simulink model "PLANTA_CONTROL_OBS"  (R2024b)
settings: Solver=FixedStepAuto  StartTime=0.0  StopTime=inf  FixedStep=0.001  MaxStep=0.0005  RelTol=1e-4
InitFcn:
  | load('ml_breakpoints.mat')
  | load('l_breakpoints.mat')
  | load('at_breakpoints.mat')
  | load('Kp_table.mat')
  | load('Kd_table.mat')
undefined symbols (not defined in the file): A_hm, A_tm, at_breakpoints, at_max, b_ha, B_hm, b_ta, B_tm, bcx, bcy, bhd, bhEb, bhm, bt, btd, btm, btw, bwu, C_hm, C_tm, D_hm, D_tm, DiscIntNeverNeededParam, dl_h_ini, dx_l_ini, dx_t_ini, dx_td_ini, dxt_max, dy_l_ini, F01_a_t_max, F01_Ts1, F02_a_h_max, F02_Ts1, F03_a_h_max, F03_a_t_max, F03_dxt_max, F03_Ts1, Fhw_min, g, Hc, ih, it, Jhd_hEb, Jhm_hb, Jtd, Jtm_tb, K_hsa, K_hsia, K_tsa, K_tsia, Kcy, Kd_table, Ke_tita, Ke_w, kp_pos, Kp_table, kp_w, Ktw, kwu, l_breakpoints ... (+26)
libraries: simulink x7, spsEdgeDetectorLib x5, simulink_extras x2, dspsigops x2, vrlib x1, dspstat3 x1
(part 3 of 4)

== system PLANTA_CONTROL_OBS/Masa contenedor ==
  Fwh : Inport
  TLK : Inport  Port=2
  Edge Detector : spsEdgeDetectorLib/Edge Detector  model=Falling  ic=0  Ts=-1
      settings: LibrarySourceBlock=sps_lib/Control/Edge Detector
  Edge Detector1 : spsEdgeDetectorLib/Edge Detector  model=Rising  ic=0  Ts=-1
      settings: LibrarySourceBlock=sps_lib/Control/Edge Detector
  Gain8 : Gain  Gain=2/g
  Product : Product
  S-R Flip-Flop : simulink_extras/Flip Flops/S-R Flip-Flop  initial_condition=0
  Unit Delay : UnitDelay  SampleTime=-1  HasFrameUpgradeWarning=on
  Mc_X : Outport
  wires:
  TLK/1 -> Unit Delay/1
  Edge Detector/1 -> S-R Flip-Flop/2
  Edge Detector1/1 -> S-R Flip-Flop/1
  S-R Flip-Flop/1 -> Product/2
  Product/1 -> Mc_X/1
  Unit Delay/1 -> Edge Detector1/1, Edge Detector/1
  Fwh/1 -> Gain8/1  "m estimada"
  Gain8/1 -> Product/1  "m estimada"

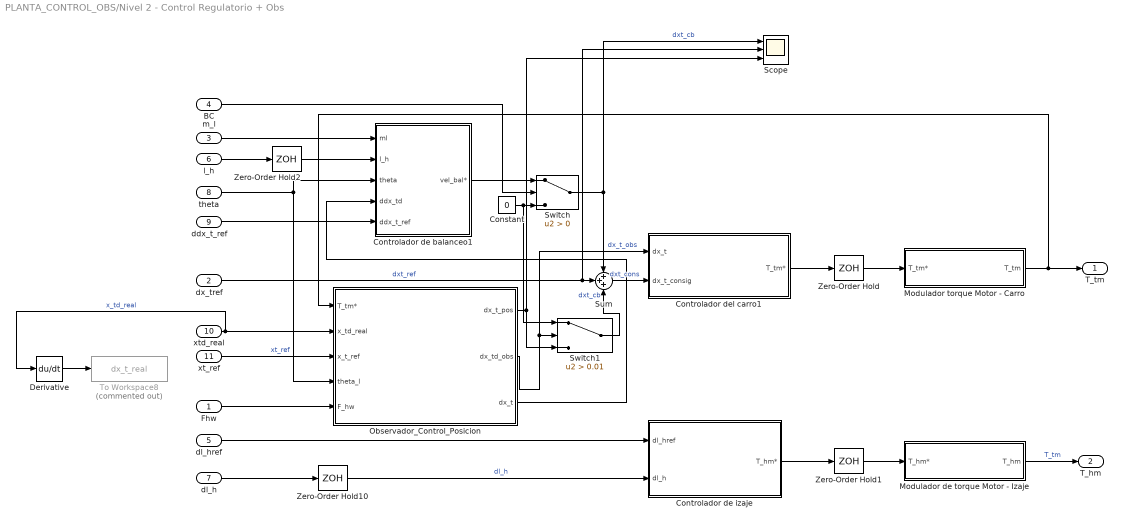
== system PLANTA_CONTROL_OBS/Nivel 2 - Control Regulatorio + Obs ==
  Fhw : Inport
  dx_tref : Inport  Port=2
  m_l : Inport  Port=3
  BC : Inport  Port=4
  dl_href : Inport  Port=5
  l_h : Inport  Port=6
  dl_h : Inport  Port=7
  theta : Inport  Port=8
  ddx_t_ref : Inport  Port=9
  xtd_real : Inport  Port=10
  xt_ref : Inport  Port=11
  Constant : Constant  Value=0
  Controlador de balanceo1 : Subsystem
  Controlador de izaje : Subsystem
  Controlador del carro1 : Subsystem
  Derivative : Derivative
  Modulador de torque Motor - Izaje : Subsystem
  Modulador torque Motor - Carro : Subsystem
  Observador_Control_Posicion : Subsystem
  Scope : Scope  NumInputPorts=3
  Sum : Sum  Inputs=+++
  Switch : Switch  Criteria=u2 > Threshold  SaturateOnIntegerOverflow=off  InputSameDT=off
  Switch1 : Switch  Criteria=u2 > Threshold  Threshold=0.01  SaturateOnIntegerOverflow=off  InputSameDT=off
  To Workspace8 : ToWorkspace  Commented=on  VariableName=dx_t_real  SaveFormat=Timeseries  SampleTime=-1
      settings: Save2DSignal=2-D array (concatenate along first dimension)
  Zero-Order Hold{,1..2,10} (4 alike) : ZeroOrderHold  SampleTime=T_s2
  T_tm : Outport
  T_hm : Outport  Port=2
  wires:
  Zero-Order Hold1/1 -> Modulador de torque Motor - Izaje/1(T_hm*)
  dl_h/1 -> Zero-Order Hold10/1
  Controlador de izaje/1(T_hm*) -> Zero-Order Hold1/1
  Modulador de torque Motor - Izaje/1(T_hm) -> T_hm/1  "T_tm"
  Zero-Order Hold/1 -> Modulador torque Motor - Carro/1(T_tm*)
  Modulador torque Motor - Carro/1(T_tm) -> Observador_Control_Posicion/1(T_tm*), T_tm/1
  l_h/1 -> Zero-Order Hold2/1
  Constant/1 -> Switch1/1, Switch/3
  m_l/1 -> Controlador de balanceo1/1(ml)
  BC/1 -> Switch/2
  Controlador del carro1/1(T_tm*) -> Zero-Order Hold/1
  Controlador de balanceo1/1(vel_bal*) -> Switch/1
  theta/1 -> Controlador de balanceo1/3(theta), Observador_Control_Posicion/4(theta_l)
  dx_tref/1 -> Scope/2, Sum/2  "dxt_ref"
  Sum/1 -> Controlador del carro1/2(dx_t_consig)  "dxt_cons"
  Switch/1 -> Scope/1, Sum/1  "dxt_cb"
  ddx_t_ref/1 -> Controlador de balanceo1/5(ddx_t_ref)
  Observador_Control_Posicion/1(dx_t_pos) -> Switch1/3, Scope/3
  xtd_real/1 -> Derivative/1, Observador_Control_Posicion/2(x_td_real)  "x_td_real"
  xt_ref/1 -> Observador_Control_Posicion/3(x_t_ref)  "xt_ref"
  Fhw/1 -> Observador_Control_Posicion/5(F_hw)
  Observador_Control_Posicion/2(dx_td_obs) -> Switch1/2, Controlador del carro1/1(dx_t)  "dx_t_obs"
  Zero-Order Hold10/1 -> Controlador de izaje/2(dl_h)  "dl_h"
  dl_href/1 -> Controlador de izaje/1(dl_href)
  Zero-Order Hold2/1 -> Controlador de balanceo1/2(l_h)
  Switch1/1 -> Sum/3  "dxt_cb"
  Derivative/1 -> To Workspace8/1
  Observador_Control_Posicion/3(dx_t) -> Controlador de balanceo1/4(ddx_td)

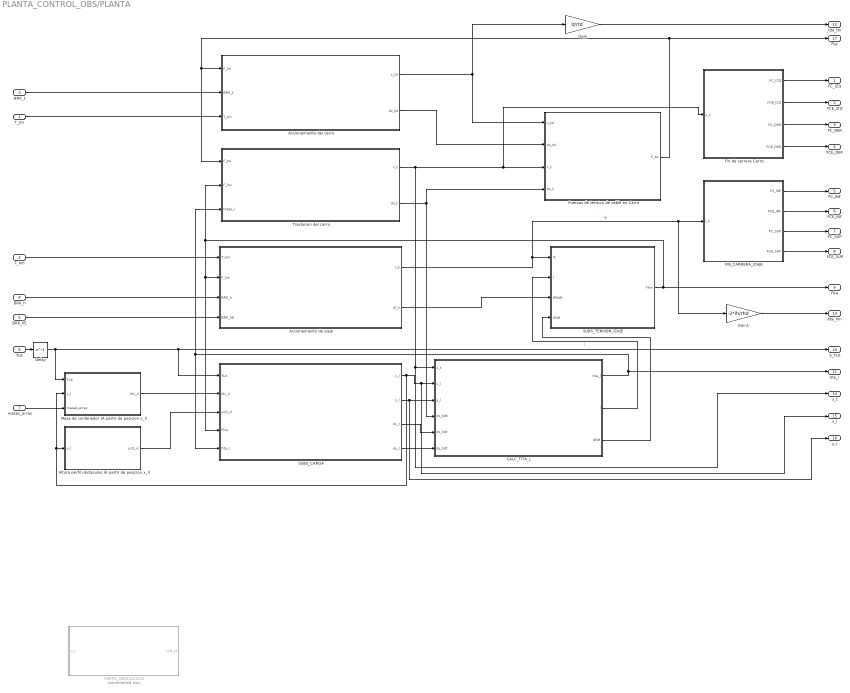
== system PLANTA_CONTROL_OBS/PLANTA ==
  T_tm : Inport
  T_hm : Inport  Port=2
  BRK_t : Inport  Port=3
  BRK_h : Inport  Port=4
  BRK_hE : Inport  Port=5
  TLK : Inport  Port=6
  masas_array : Inport  Port=7
  Accionamiento de Izaje : Subsystem
  Accionamiento del carro : Subsystem
  Altura perfil obstaculos (A partir de posicion x_l) : Subsystem
  CALC_TITA_L : Subsystem
  Delay : Delay  DelayLength=1  InputProcessing=Columns as channels (frame based)  SampleTime=T_s1
  FIN_CARRERA_IZAJE : Subsystem
  Fin de carrera Carro : Subsystem
  Fuerzas de tension de cable en Carro : Subsystem
  Gain : Gain  Gain=it/rtd
  Gain1 : Gain  Gain=-2*ih/rhd
  Masa de contenedor (A partir de posicion x_l) : Subsystem
  PERFIL_OBSTACULOS : Subsystem  Commented=on
  SUBS_CARGA : Subsystem
  SUBS_TENSION_IZAJE : Subsystem
  Traslacion del carro : Subsystem
  FC_IZQ : Outport
  FCE_IZQ : Outport  Port=2
  FC_DER : Outport  Port=3
  FCE_DER : Outport  Port=4
  FC_INF : Outport  Port=5
  FCE_INF : Outport  Port=6
  FC_SUP : Outport  Port=7
  FCE_SUP : Outport  Port=8
  Fhw : Outport  Port=9
  S_TLK : Outport  Port=10
  tita_l : Outport  Port=11
  tita_tm : Outport  Port=12
  tita_hm : Outport  Port=13
  x_t : Outport  Port=14
  x_l : Outport  Port=15
  y_l : Outport  Port=16
  Ftw : Outport  Port=17
  wires:
  Gain/1 -> tita_tm/1
  Traslacion del carro/2(dx_t) -> CALC_TITA_L/4(dx_t/dt), Fuerzas de tension de cable en Carro/4(dx_t)
  SUBS_TENSION_IZAJE/1(Fhw) -> Fhw/1, Traslacion del carro/2(F_hw), Accionamiento de Izaje/2(F_hw), SUBS_CARGA/4(Fhw)
  CALC_TITA_L/3(dl/dt) -> SUBS_TENSION_IZAJE/4(dl/dt)
  BRK_h/1 -> Accionamiento de Izaje/3(BRK_h)
  TLK/1 -> Delay/1
  BRK_t/1 -> Accionamiento del carro/2(BRK_t)
  Accionamiento del carro/1(x_td) -> Gain/1, Fuerzas de tension de cable en Carro/1(x_td)
  BRK_hE/1 -> Accionamiento de Izaje/4(BRK_hE)
  Accionamiento del carro/2(dx_td) -> Fuerzas de tension de cable en Carro/2(dx_td)
  FIN_CARRERA_IZAJE/3(FC_SUP) -> FC_SUP/1
  Fin de carrera Carro/4(FCE_DER) -> FCE_DER/1
  SUBS_CARGA/4(dy_l) -> CALC_TITA_L/6(dy_l/dt)
  CALC_TITA_L/2(l) -> SUBS_TENSION_IZAJE/2(l)  "l"
  Fuerzas de tension de cable en Carro/1(F_tw) -> Ftw/1, Accionamiento del carro/1(F_tw), Traslacion del carro/1(F_tw)
  SUBS_CARGA/3(dx_l) -> CALC_TITA_L/5(dx_l/dt)
  Altura perfil obstaculos (A partir de posicion x_l)/1(yc0_xl) -> SUBS_CARGA/3(yc0_xl)
  Accionamiento de Izaje/1(l_h) -> SUBS_TENSION_IZAJE/1(Ih), FIN_CARRERA_IZAJE/1(l_h), Gain1/1  "lh"
  Accionamiento de Izaje/2(dl_h) -> SUBS_TENSION_IZAJE/3(dlh/dt)
  T_tm/1 -> Accionamiento del carro/3(T_tm)
  Fin de carrera Carro/2(FCE_IZQ) -> FCE_IZQ/1
  T_hm/1 -> Accionamiento de Izaje/1(T_hm)
  FIN_CARRERA_IZAJE/1(FC_INF) -> FC_INF/1
  Gain1/1 -> tita_hm/1
  FIN_CARRERA_IZAJE/2(FCE_INF) -> FCE_INF/1
  Fin de carrera Carro/1(FC_IZQ) -> FC_IZQ/1
  FIN_CARRERA_IZAJE/4(FCE_SUP) -> FCE_SUP/1
  Fin de carrera Carro/3(FC_DER) -> FC_DER/1
  SUBS_CARGA/1(x_l) -> Masa de contenedor (A partir de posicion x_l)/2(x_l), Altura perfil obstaculos (A partir de posicion x_l)/1(x_l), x_l/1, CALC_TITA_L/2(x_l)
  CALC_TITA_L/1(tita_l) -> tita_l/1, Traslacion del carro/3(theta_l), SUBS_CARGA/5(tita_l)
  Traslacion del carro/1(x_t) -> CALC_TITA_L/1(x_t), x_t/1, Fin de carrera Carro/1(x_t), Fuerzas de tension de cable en Carro/3(x_t)
  SUBS_CARGA/2(y_l) -> y_l/1, CALC_TITA_L/3(y_l)
  Masa de contenedor (A partir de posicion x_l)/1(Mc_X) -> SUBS_CARGA/2(Mc_X)
  Delay/1 -> Masa de contenedor (A partir de posicion x_l)/1(TLK), S_TLK/1, SUBS_CARGA/1(TLK)
  masas_array/1 -> Masa de contenedor (A partir de posicion x_l)/3(masas_array)

== system PLANTA_CONTROL_OBS/Actualizar perfil/Enabled Subsystem ==
  index : Inport
  Enable : EnablePort
  Actualiza perfil : MATLAB Function  TreatAsAtomicUnit=on
  Constant16 : Constant  Value=Hc
  Data Store Read3 : DataStoreRead  DataStoreName=y0_global  IndexOptions=Index vector (dialog)  Indices=1  OutputSizes=1
  y0_actualizado : Outport
  wires:
  Data Store Read3/1 -> Actualiza perfil/2(y0)
  Constant16/1 -> Actualiza perfil/3(Hc)
  index/1 -> Actualiza perfil/1(index)
  Actualiza perfil/1(y0_actualizado) -> y0_actualizado/1

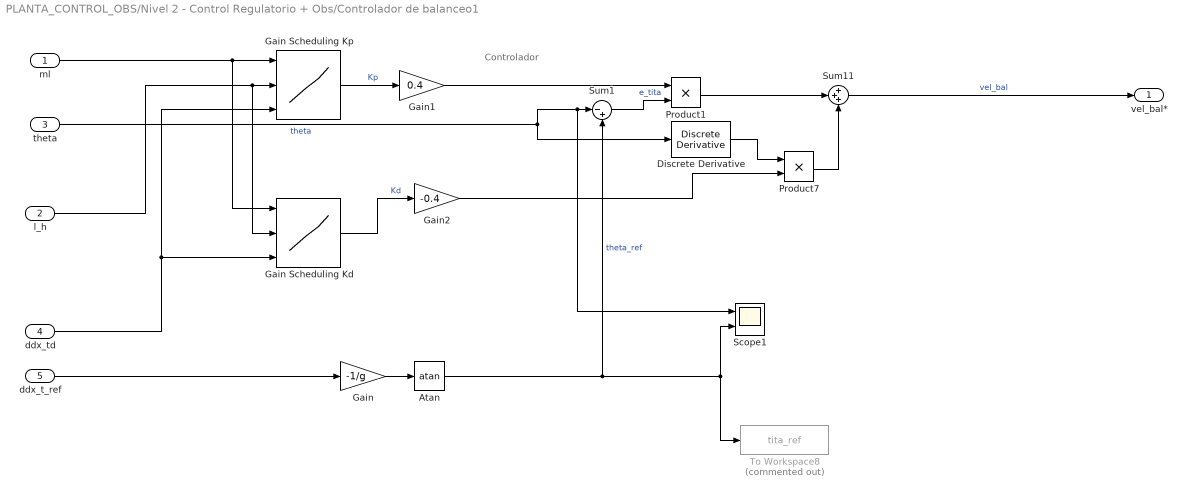
== system PLANTA_CONTROL_OBS/Nivel 2 - Control Regulatorio + Obs/Controlador de balanceo1 ==
  note: Controlador
  ml : Inport
  l_h : Inport  Port=2
  theta : Inport  Port=3
  ddx_td : Inport  Port=4
  ddx_t_ref : Inport  Port=5
  Atan : Trigonometry  Operator=atan
  Discrete Derivative : simulink/Discrete/Discrete Derivative  gainval=1.0  ICPrevScaledInput=0.0  OutMin=[]  OutMax=[]  OutDataType=fixdt(1, 16)  OutScaling=2^-10  DoSatur=off
  Gain : Gain  Gain=-1/g
  Gain Scheduling Kd : Lookup_n-D  NumberOfTableDimensions=3  BreakpointsForDimension1=ml_breakpoints  BreakpointsForDimension2=l_breakpoints  BreakpointsForDimension3=at_breakpoints  BreakpointsForDimension4=at_breakpoints  Table=Kd_table  InterpMethod=Flat  ExtrapMethod=Clip  InternalRulePriority=Speed  RndMeth=Simplest
      settings: InputPortMap=u0,u1,u2
  Gain Scheduling Kp : Lookup_n-D  NumberOfTableDimensions=3  BreakpointsForDimension1=ml_breakpoints  BreakpointsForDimension2=l_breakpoints  BreakpointsForDimension3=at_breakpoints  BreakpointsForDimension4=at_breakpoints  Table=Kp_table  InterpMethod=Flat  ExtrapMethod=Clip  InternalRulePriority=Speed  RndMeth=Simplest
      settings: InputPortMap=u0,u1,u2
  Gain1 : Gain  Gain=0.4
  Gain2 : Gain  Gain=-0.4
  Product1 : Product
  Product7 : Product
  Scope1 : Scope  NumInputPorts=2
  Sum1 : Sum  Inputs=|-+
  Sum11 : Sum  Inputs=+++
  To Workspace8 : ToWorkspace  Commented=on  VariableName=tita_ref  SaveFormat=Timeseries  SampleTime=-1
      settings: Save2DSignal=2-D array (concatenate along first dimension)
  vel_bal* : Outport
  wires:
  Discrete Derivative/1 -> Product7/1
  Gain Scheduling Kd/1 -> Gain2/1  "Kd"
  Gain/1 -> Atan/1
  Gain Scheduling Kp/1 -> Gain1/1  "Kp"
  theta/1 -> Scope1/1, Sum1/1, Discrete Derivative/1  "theta"
  Product1/1 -> Sum11/2
  Atan/1 -> To Workspace8/1, Scope1/2, Sum1/2  "theta_ref"
  Product7/1 -> Sum11/3
  ddx_t_ref/1 -> Gain/1
  Sum1/1 -> Product1/2  "e_tita"
  Sum11/1 -> vel_bal*/1  "vel_bal"
  ml/1 -> Gain Scheduling Kd/1, Gain Scheduling Kp/1
  l_h/1 -> Gain Scheduling Kd/2, Gain Scheduling Kp/2
  Gain1/1 -> Product1/1
  Gain2/1 -> Product7/2
  ddx_td/1 -> Gain Scheduling Kd/3, Gain Scheduling Kp/3

== system PLANTA_CONTROL_OBS/Nivel 2 - Control Regulatorio + Obs/Controlador de izaje ==
  dl_href : Inport
  dl_h : Inport  Port=2
  Discrete-Time Integrator : DiscreteIntegrator  SampleTime=T_s2  ICPrevOutput=DiscIntNeverNeededParam  ICPrevScaledInput=DiscIntNeverNeededParam
  Discrete-Time Integrator1 : DiscreteIntegrator  SampleTime=T_s2  ICPrevOutput=DiscIntNeverNeededParam  ICPrevScaledInput=DiscIntNeverNeededParam
  Gain1 : Gain  Gain=K_hsia
  Gain2 : Gain  Gain=b_ha
  Gain8 : Gain  Gain=K_hsa
  Sum : Sum  Inputs=|+-
  Sum5 : Sum  Inputs=+|+|+
  T_hm* : Outport
  wires:
  Gain2/1 -> Sum5/3
  dl_h/1 -> Sum/2
  Sum5/1 -> T_hm*/1
  dl_href/1 -> Sum/1
  Gain1/1 -> Sum5/1
  Sum/1 -> Gain2/1, Discrete-Time Integrator/1  "d_ek"
  Gain8/1 -> Sum5/2
  Discrete-Time Integrator/1 -> Gain8/1, Discrete-Time Integrator1/1
  Discrete-Time Integrator1/1 -> Gain1/1

== system PLANTA_CONTROL_OBS/Nivel 2 - Control Regulatorio + Obs/Controlador del carro1 ==
  dx_t : Inport
  dx_t_consig : Inport  Port=2
  Discrete-Time Integrator : DiscreteIntegrator  SampleTime=T_s2  ICPrevOutput=DiscIntNeverNeededParam  ICPrevScaledInput=DiscIntNeverNeededParam
  Discrete-Time Integrator1 : DiscreteIntegrator  SampleTime=T_s2  ICPrevOutput=DiscIntNeverNeededParam  ICPrevScaledInput=DiscIntNeverNeededParam
  Gain1 : Gain  Gain=b_ta
  Gain2 : Gain  Gain=K_tsa
  Gain4 : Gain  Gain=K_tsia
  Sum : Sum  Inputs=|+-
  Sum5 : Sum  Inputs=+|+|+
  T_tm* : Outport
  wires:
  Sum/1 -> Discrete-Time Integrator/1, Gain1/1  "d_ek"
  dx_t_consig/1 -> Sum/1
  Sum5/1 -> T_tm*/1
  dx_t/1 -> Sum/2
  Gain2/1 -> Sum5/2
  Gain1/1 -> Sum5/3
  Gain4/1 -> Sum5/1
  Discrete-Time Integrator/1 -> Gain2/1, Discrete-Time Integrator1/1
  Discrete-Time Integrator1/1 -> Gain4/1

== system PLANTA_CONTROL_OBS/Nivel 2 - Control Regulatorio + Obs/Modulador de torque Motor - Izaje ==
  T_hm* : Inport
  State-Space : StateSpace  A=A_hm  B=B_hm  C=C_hm  D=D_hm  InitialCondition=0
  T_hm : Outport
  wires:
  T_hm*/1 -> State-Space/1
  State-Space/1 -> T_hm/1

== system PLANTA_CONTROL_OBS/Nivel 2 - Control Regulatorio + Obs/Modulador torque Motor - Carro ==
  T_tm* : Inport
  State-Space : StateSpace  A=A_tm  B=B_tm  C=C_tm  D=D_tm  InitialCondition=0
  T_tm : Outport
  wires:
  State-Space/1 -> T_tm/1
  T_tm*/1 -> State-Space/1

== system PLANTA_CONTROL_OBS/Nivel 2 - Control Regulatorio + Obs/Observador_Control_Posicion ==
  T_tm* : Inport
  x_td_real : Inport  Port=2
  x_t_ref : Inport  Port=3
  theta_l : Inport  Port=4
  F_hw : Inport  Port=5
  Discrete Derivative : simulink/Discrete/Discrete Derivative  gainval=1.0  ICPrevScaledInput=0.0  OutMin=[]  OutMax=[]  OutDataType=fixdt(1, 16)  OutScaling=2^-10  DoSatur=off
  Fuerzas de tension de cable en Carro : Subsystem
  Observador : Subsystem
  Subsystem : Subsystem
  Traslacion del carro : Subsystem
  dx_t_pos : Outport
  dx_td_obs : Outport  Port=2
  dx_t : Outport  Port=3
  wires:
  Observador/1(dx_td_obs) -> Fuerzas de tension de cable en Carro/2(dx_td), dx_td_obs/1  "dx_td_obs"
  x_td_real/1 -> Fuerzas de tension de cable en Carro/1(x_td), Observador/1(x_td)
  x_t_ref/1 -> Subsystem/2(xt_ref)
  Subsystem/1(dxt_pos) -> dx_t_pos/1
  Traslacion del carro/1(x_t) -> Fuerzas de tension de cable en Carro/3(x_t), Subsystem/1(xt_obs)  "x_t_obs"
  Traslacion del carro/2(dx_t) -> Fuerzas de tension de cable en Carro/4(dx_t), Discrete Derivative/1  "dx_t_obs"
  theta_l/1 -> Traslacion del carro/3(theta_l)
  F_hw/1 -> Traslacion del carro/2(F_hw)
  Fuerzas de tension de cable en Carro/1(F_tw) -> Traslacion del carro/1(F_tw)
  T_tm*/1 -> Observador/2(T_tm*)
  Discrete Derivative/1 -> dx_t/1

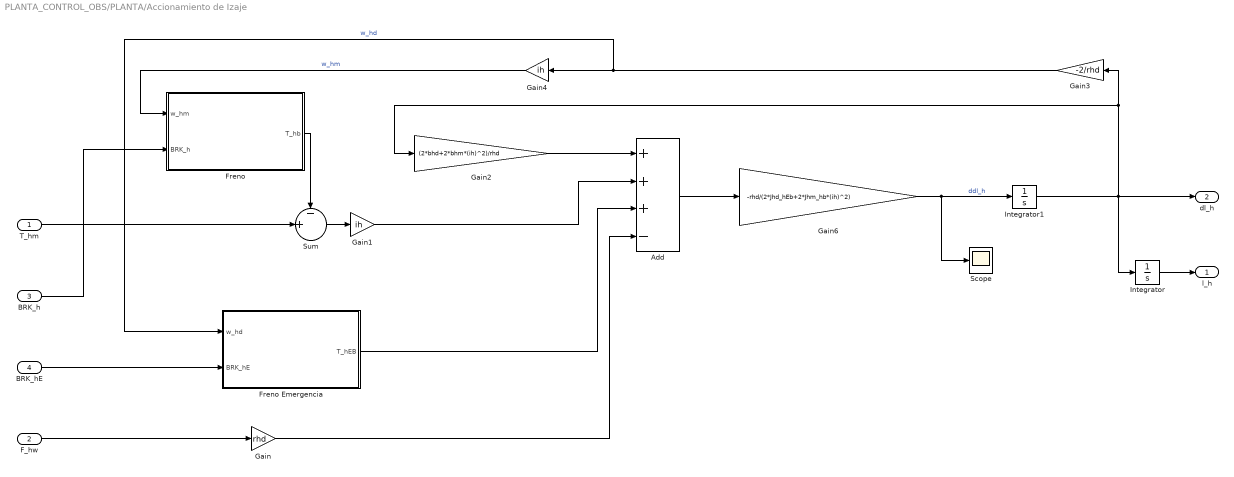
== system PLANTA_CONTROL_OBS/PLANTA/Accionamiento de Izaje ==
  T_hm : Inport
  F_hw : Inport  Port=2
  BRK_h : Inport  Port=3
  BRK_hE : Inport  Port=4
  Add : Sum  Inputs=+++-
  Freno : Subsystem
  Freno Emergencia : Subsystem
  Gain : Gain  Gain=rhd
  Gain1 : Gain  Gain=ih
  Gain2 : Gain  Gain=(2*bhd+2*bhm*(ih)^2)/rhd
  Gain3 : Gain  Gain=-2/rhd
  Gain4 : Gain  Gain=ih
  Gain6 : Gain  Gain=-rhd/(2*Jhd_hEb+2*Jhm_hb*(ih)^2)
  Integrator : Integrator  InitialCondition=l_h_ini
  Integrator1 : Integrator  InitialCondition=dl_h_ini
  Scope : Scope
  Sum : Sum  Inputs=-|+||
  l_h : Outport
  dl_h : Outport  Port=2
  wires:
  Gain1/1 -> Add/2
  Integrator1/1 -> dl_h/1, Integrator/1, Gain3/1, Gain2/1
  F_hw/1 -> Gain/1
  Gain6/1 -> Scope/1, Integrator1/1  "ddl_h"
  T_hm/1 -> Sum/2
  Freno Emergencia/1(T_hEB) -> Add/3
  BRK_hE/1 -> Freno Emergencia/2(BRK_hE)
  Gain4/1 -> Freno/1(w_hm)  "w_hm"
  Gain/1 -> Add/4
  Integrator/1 -> l_h/1
  Gain3/1 -> Freno Emergencia/1(w_hd), Gain4/1  "w_hd"
  Sum/1 -> Gain1/1
  Add/1 -> Gain6/1
  Freno/1(T_hb) -> Sum/1
  Gain2/1 -> Add/1
  BRK_h/1 -> Freno/2(BRK_h)

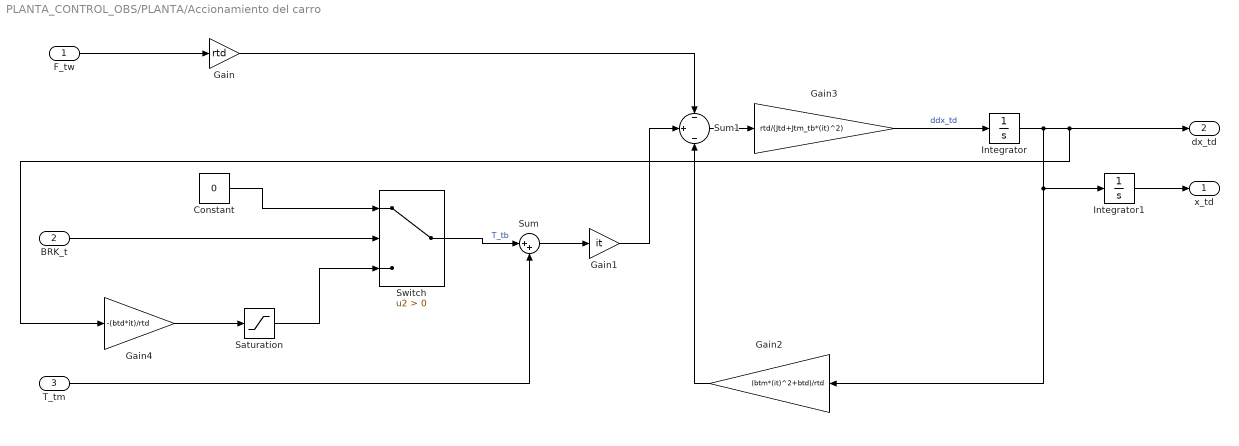
== system PLANTA_CONTROL_OBS/PLANTA/Accionamiento del carro ==
  F_tw : Inport
  BRK_t : Inport  Port=2
  T_tm : Inport  Port=3
  Constant : Constant  Value=0
  Gain : Gain  Gain=rtd
  Gain1 : Gain  Gain=it
  Gain2 : Gain  Gain=(btm*(it)^2+btd)/rtd
  Gain3 : Gain  Gain=rtd/(Jtd+Jtm_tb*(it)^2)
  Gain4 : Gain  Gain=-(btd*it)/rtd
  Integrator : Integrator  InitialCondition=dx_td_ini
  Integrator1 : Integrator  InitialCondition=x_td_ini
  Saturation : Saturate  UpperLimit=Ttb_Max  LowerLimit=-Ttb_Max
  Sum : Sum  Inputs=|++
  Sum1 : Sum  Inputs=-|+|-
  Switch : Switch  Criteria=u2 > Threshold  SaturateOnIntegerOverflow=off  InputSameDT=off
  x_td : Outport
  dx_td : Outport  Port=2
  wires:
  Integrator/1 -> Gain4/1, dx_td/1, Integrator1/1, Gain2/1
  Gain4/1 -> Saturation/1
  T_tm/1 -> Sum/2
  Constant/1 -> Switch/1
  Gain/1 -> Sum1/1
  Saturation/1 -> Switch/3
  Gain3/1 -> Integrator/1  "ddx_td"
  BRK_t/1 -> Switch/2
  Sum1/1 -> Gain3/1
  Switch/1 -> Sum/1  "T_tb"
  F_tw/1 -> Gain/1
  Gain1/1 -> Sum1/2
  Integrator1/1 -> x_td/1
  Gain2/1 -> Sum1/3
  Sum/1 -> Gain1/1

== system PLANTA_CONTROL_OBS/PLANTA/Altura perfil obstaculos (A partir de posicion x_l) ==
  x_l : Inport
  Ajuste referencia : Constant  Value=30
  Calculo : MATLAB Function  TreatAsAtomicUnit=on
  Data Store Read : DataStoreRead  DataStoreName=y0_global  IndexOptions=Index vector (dialog)  Indices=1  OutputSizes=1
  Data Type Conversion : DataTypeConversion  OutDataTypeStr=int32  RndMeth=Ceiling  SaturateOnIntegerOverflow=off
  Gain1 : Gain  Gain=1/Wc
  Scope : Scope
  Scope1 : Scope
  Sum : Sum  Inputs=|++
  yc0_xl : Outport
  wires:
  Calculo/1(yc0_xt) -> Scope1/1, yc0_xl/1
  Data Store Read/1 -> Calculo/1(y0_array)
  Data Type Conversion/1 -> Scope/1, Calculo/2(index)
  Gain1/1 -> Data Type Conversion/1
  Ajuste referencia/1 -> Sum/2
  Sum/1 -> Gain1/1
  x_l/1 -> Sum/1

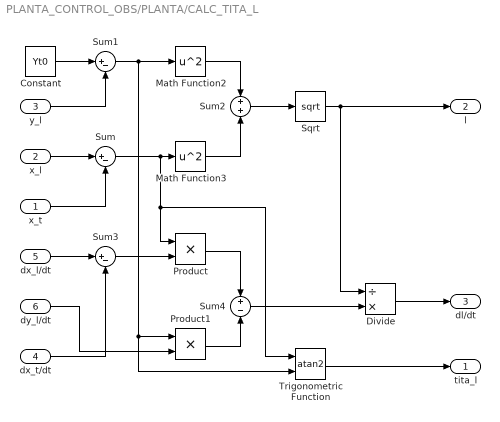
== system PLANTA_CONTROL_OBS/PLANTA/CALC_TITA_L ==
  x_t : Inport
  x_l : Inport  Port=2
  y_l : Inport  Port=3
  dx_t/dt : Inport  Port=4
  dx_l/dt : Inport  Port=5
  dy_l/dt : Inport  Port=6
  Constant : Constant  Value=Yt0
  Divide : Product  Inputs=/*
  Math Function2 : Math  Operator=square
  Math Function3 : Math  Operator=square
  Product : Product
  Product1 : Product
  Sqrt : Sqrt
  Sum : Sum  Inputs=|+-
  Sum1 : Sum  Inputs=|+-
  Sum2 : Sum  Inputs=+|+
  Sum3 : Sum  Inputs=|+-
  Sum4 : Sum  Inputs=+|-
  Trigonometric Function : Trigonometry  Operator=atan2
  tita_l : Outport
  l : Outport  Port=2
  dl/dt : Outport  Port=3
  wires:
  Product/1 -> Sum4/1
  Product1/1 -> Sum4/2
  x_l/1 -> Sum/1
  dx_t/dt/1 -> Sum3/2
  y_l/1 -> Sum1/2
  Sum/1 -> Product/1, Trigonometric Function/1, Math Function3/1
  Sqrt/1 -> l/1, Divide/1
  Sum2/1 -> Sqrt/1
  Sum4/1 -> Divide/2
  Sum1/1 -> Product1/1, Trigonometric Function/2, Math Function2/1
  Math Function2/1 -> Sum2/1
  dx_l/dt/1 -> Sum3/1
  x_t/1 -> Sum/2
  Constant/1 -> Sum1/1
  Sum3/1 -> Product/2
  dy_l/dt/1 -> Product1/2
  Math Function3/1 -> Sum2/2
  Trigonometric Function/1 -> tita_l/1
  Divide/1 -> dl/dt/1

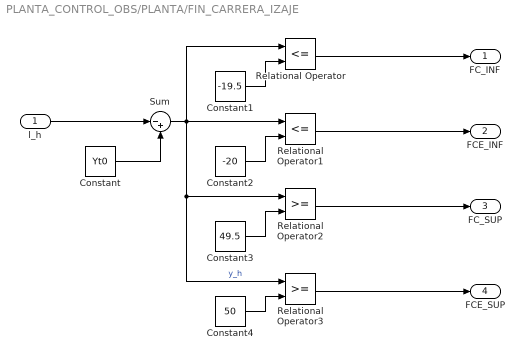
== system PLANTA_CONTROL_OBS/PLANTA/FIN_CARRERA_IZAJE ==
  l_h : Inport
  Constant : Constant  Value=Yt0
  Constant1 : Constant  Value=-19.5
  Constant2 : Constant  Value=-20
  Constant3 : Constant  Value=49.5
  Constant4 : Constant  Value=50
  Relational Operator : RelationalOperator  Operator=<=  OutDataTypeStr=boolean  RndMeth=Simplest  InputSameDT=off
  Relational Operator1 : RelationalOperator  Operator=<=  OutDataTypeStr=boolean  RndMeth=Simplest  InputSameDT=off
  Relational Operator2 : RelationalOperator  OutDataTypeStr=boolean  RndMeth=Simplest  InputSameDT=off
  Relational Operator3 : RelationalOperator  OutDataTypeStr=boolean  RndMeth=Simplest  InputSameDT=off
  Sum : Sum  Inputs=|-+
  FC_INF : Outport
  FCE_INF : Outport  Port=2
  FC_SUP : Outport  Port=3
  FCE_SUP : Outport  Port=4
  wires:
  Sum/1 -> Relational Operator3/1, Relational Operator2/1, Relational Operator/1, Relational Operator1/1  "y_h"
  Relational Operator3/1 -> FCE_SUP/1
  Constant4/1 -> Relational Operator3/2
  Relational Operator2/1 -> FC_SUP/1
  Constant3/1 -> Relational Operator2/2
  Constant1/1 -> Relational Operator/2
  Constant2/1 -> Relational Operator1/2
  Relational Operator/1 -> FC_INF/1
  Constant/1 -> Sum/2
  Relational Operator1/1 -> FCE_INF/1
  l_h/1 -> Sum/1

== system PLANTA_CONTROL_OBS/PLANTA/Fin de carrera Carro ==
  x_t : Inport
  Constant : Constant  Value=-29.5
  Constant1 : Constant  Value=-30
  Constant2 : Constant  Value=49.5
  Constant3 : Constant  Value=50
  Relational Operator : RelationalOperator  Operator=<=  OutDataTypeStr=boolean  RndMeth=Simplest  InputSameDT=off
  Relational Operator1 : RelationalOperator  Operator=<=  OutDataTypeStr=boolean  RndMeth=Simplest  InputSameDT=off
  Relational Operator2 : RelationalOperator  OutDataTypeStr=boolean  RndMeth=Simplest  InputSameDT=off
  Relational Operator3 : RelationalOperator  OutDataTypeStr=boolean  RndMeth=Simplest  InputSameDT=off
  FC_IZQ : Outport
  FCE_IZQ : Outport  Port=2
  FC_DER : Outport  Port=3
  FCE_DER : Outport  Port=4
  wires:
  Relational Operator/1 -> FC_IZQ/1
  Constant1/1 -> Relational Operator1/2
  x_t/1 -> Relational Operator3/1, Relational Operator2/1, Relational Operator/1, Relational Operator1/1
  Relational Operator1/1 -> FCE_IZQ/1
  Constant2/1 -> Relational Operator2/2
  Relational Operator2/1 -> FC_DER/1
  Relational Operator3/1 -> FCE_DER/1
  Constant3/1 -> Relational Operator3/2
  Constant/1 -> Relational Operator/2

== system PLANTA_CONTROL_OBS/PLANTA/Fuerzas de tension de cable en Carro ==
  x_td : Inport
  dx_td : Inport  Port=2
  x_t : Inport  Port=3
  dx_t : Inport  Port=4
  Add : Sum  Inputs=+-
  Add1 : Sum  Inputs=+-
  Add2 : Sum
  Gain : Gain  Gain=Ktw
  Gain1 : Gain  Gain=btw
  F_tw : Outport
  wires:
  Add1/1 -> Gain1/1
  Add/1 -> Gain/1
  Gain1/1 -> Add2/2
  x_td/1 -> Add/1
  dx_t/1 -> Add1/2
  dx_td/1 -> Add1/1
  Gain/1 -> Add2/1
  Add2/1 -> F_tw/1
  x_t/1 -> Add/2

== system PLANTA_CONTROL_OBS/PLANTA/Masa de contenedor (A partir de posicion x_l) ==
  TLK : Inport
  x_l : Inport  Port=2
  masas_array : Inport  Port=3
  Ajuste referencia : Constant  Value=30
  Calculo : MATLAB Function  TreatAsAtomicUnit=on
  Data Type Conversion : DataTypeConversion  OutDataTypeStr=int32  RndMeth=Ceiling  SaturateOnIntegerOverflow=off
  Edge Detector : spsEdgeDetectorLib/Edge Detector  model=Falling  ic=0  Ts=-1
  Edge Detector1 : spsEdgeDetectorLib/Edge Detector  model=Rising  ic=0  Ts=-1
  Gain1 : Gain  Gain=1/Wc
  Product : Product
  S-R Flip-Flop : simulink_extras/Flip Flops/S-R Flip-Flop  initial_condition=0
  Sample and Hold : dspsigops/Sample and Hold  trig=Rising edge  initCond=0  latchinput=off
  Sum : Sum  Inputs=|++
  Unit Delay : UnitDelay  SampleTime=-1  HasFrameUpgradeWarning=on
  Mc_X : Outport
  wires:
  Data Type Conversion/1 -> Calculo/2(index)
  Gain1/1 -> Data Type Conversion/1
  Ajuste referencia/1 -> Sum/2
  Sum/1 -> Gain1/1
  x_l/1 -> Sum/1
  TLK/1 -> Unit Delay/1
  Edge Detector/1 -> S-R Flip-Flop/2
  Edge Detector1/1 -> S-R Flip-Flop/1
  S-R Flip-Flop/1 -> Sample and Hold/Trigger, Product/2
  Product/1 -> Mc_X/1
  Unit Delay/1 -> Edge Detector1/1, Edge Detector/1
  Calculo/1(Mc_X) -> Sample and Hold/1
  Sample and Hold/1 -> Product/1
  masas_array/1 -> Calculo/1(masas_array)

== system PLANTA_CONTROL_OBS/PLANTA/PERFIL_OBSTACULOS ==
  note: LIDAR
  x_t : Inport
  Ajuste distancia LIDAR : dspsigops/Variable Fractional Delay  mode=OBSOLETE  modeActive=Linear  L=4  FarrowL=4  R=10  alpha=1  dmax=100  InputProcessing=Columns as channels (frame based)  ic=0  noDFT=off  fallbackFIR=Clip to the minimum value necessary for centered kernel  fallbackFarrow=Clip to the minimum value necessary for centered kernel  roundingMode=Zero  overflowMode=off
  Ajuste referencia : Constant  Value=30
  Constant : Constant  Value=Yt0
  Data Type Conversion : DataTypeConversion  OutDataTypeStr=int32  RndMeth=Ceiling  SaturateOnIntegerOverflow=off
  Delay : Delay  DelayLength=1  InputProcessing=Columns as channels (frame based)  SampleTime=0.001
  Delay espacial : Constant  Value=3/Wc
  Gain : Gain  Gain=1/Wc
  Perfil obstaculos (ENTORNO) : FromWorkspace  VariableName=y0
  Posicion LIDAR : Constant  Value=3
  Sum : Sum  Inputs=|++
  Sum1 : Sum  Inputs=|++
  Sum2 : Sum  Inputs=+-|
  sensor : MATLAB Function  TreatAsAtomicUnit=on
  yc0_xt : Outport
  wires:
  Delay/1 -> Sum1/1
  Sum/1 -> Gain/1
  Constant/1 -> Sum2/1
  Sum2/1 -> yc0_xt/1
  Sum1/1 -> Sum/1
  Delay espacial/1 -> Ajuste distancia LIDAR/2
  Ajuste distancia LIDAR/1 -> Sum2/2
  Data Type Conversion/1 -> sensor/2(index)
  Perfil obstaculos (ENTORNO)/1 -> sensor/1(y0_array)
  sensor/1(distancia) -> Ajuste distancia LIDAR/1
  Posicion LIDAR/1 -> Sum1/2
  Gain/1 -> Data Type Conversion/1
  x_t/1 -> Delay/1
  Ajuste referencia/1 -> Sum/2

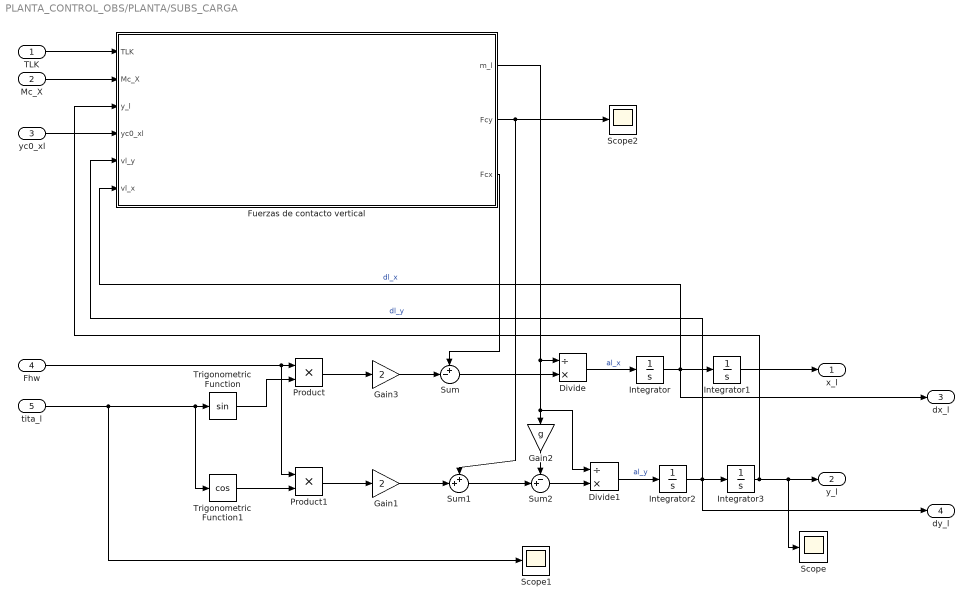
== system PLANTA_CONTROL_OBS/PLANTA/SUBS_CARGA ==
  TLK : Inport
  Mc_X : Inport  Port=2
  yc0_xl : Inport  Port=3
  Fhw : Inport  Port=4
  tita_l : Inport  Port=5
  Divide : Product  Inputs=/*
  Divide1 : Product  Inputs=/*
  Fuerzas de contacto vertical : Subsystem
  Gain1 : Gain  Gain=2
  Gain2 : Gain  Gain=g
  Gain3 : Gain  Gain=2
  Integrator : Integrator  InitialCondition=dx_l_ini  AbsoluteTolerance=-1
  Integrator1 : Integrator  InitialCondition=x_l_ini
  Integrator2 : Integrator  InitialCondition=dy_l_ini
  Integrator3 : Integrator  InitialCondition=y_l_ini
  Product : Product
  Product1 : Product
  Scope : Scope
  Scope1 : Scope
  Scope2 : Scope
  Sum : Sum  Inputs=+-|
  Sum1 : Sum  Inputs=++|
  Sum2 : Sum  Inputs=-+|
  Trigonometric Function : Trigonometry
  Trigonometric Function1 : Trigonometry  Operator=cos
  x_l : Outport
  y_l : Outport  Port=2
  dx_l : Outport  Port=3
  dy_l : Outport  Port=4
  wires:
  Divide1/1 -> Integrator2/1  "al_y"
  Sum2/1 -> Divide1/2
  Integrator2/1 -> dy_l/1, Integrator3/1, Fuerzas de contacto vertical/5(vl_y)  "dl_y"
  Fhw/1 -> Product1/1, Product/1
  Integrator3/1 -> Scope/1, y_l/1, Fuerzas de contacto vertical/3(y_l)
  Divide/1 -> Integrator/1  "al_x"
  Product1/1 -> Gain1/1
  Sum/1 -> Divide/2
  Fuerzas de contacto vertical/1(m_l) -> Divide/1, Divide1/1, Gain2/1
  Gain1/1 -> Sum1/2
  Trigonometric Function1/1 -> Product1/2
  Fuerzas de contacto vertical/3(Fcx) -> Sum/1
  Gain2/1 -> Sum2/1
  Integrator/1 -> dx_l/1, Fuerzas de contacto vertical/6(vl_x), Integrator1/1  "dl_x"
  Fuerzas de contacto vertical/2(Fcy) -> Sum1/1, Scope2/1
  tita_l/1 -> Scope1/1, Trigonometric Function1/1, Trigonometric Function/1
  Product/1 -> Gain3/1
  yc0_xl/1 -> Fuerzas de contacto vertical/4(yc0_xl)
  Trigonometric Function/1 -> Product/2
  Integrator1/1 -> x_l/1
  Sum1/1 -> Sum2/2
  Gain3/1 -> Sum/2
  Mc_X/1 -> Fuerzas de contacto vertical/2(Mc_X)
  TLK/1 -> Fuerzas de contacto vertical/1(TLK)

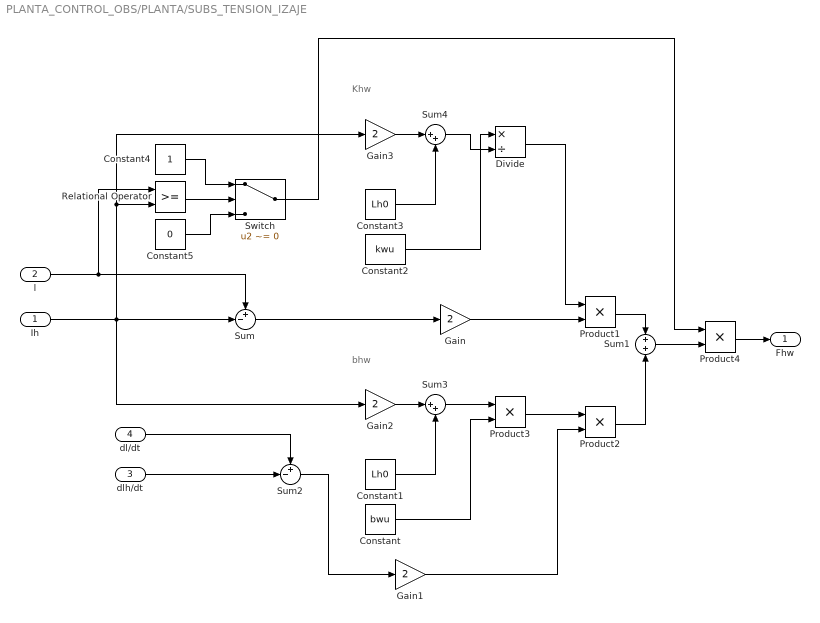
== system PLANTA_CONTROL_OBS/PLANTA/SUBS_TENSION_IZAJE ==
  note: Khw
  note: bhw
  Ih : Inport
  l : Inport  Port=2
  dlh/dt : Inport  Port=3
  dl/dt : Inport  Port=4
  Constant : Constant  Value=bwu
  Constant1 : Constant  Value=Lh0
  Constant2 : Constant  Value=kwu
  Constant3 : Constant  Value=Lh0
  Constant4 : Constant  OutDataTypeStr=double
  Constant5 : Constant  Value=0  OutDataTypeStr=double
  Divide : Product  Inputs=*/
  Gain : Gain  Gain=2
  Gain1 : Gain  Gain=2
  Gain2 : Gain  Gain=2  OutDataTypeStr=Inherit: Inherit via back propagation
  Gain3 : Gain  Gain=2  OutDataTypeStr=Inherit: Inherit via back propagation
  Product{1..4} (4 alike) : Product
  Relational Operator : RelationalOperator  OutDataTypeStr=boolean  RndMeth=Simplest  InputSameDT=off
  Sum : Sum  Inputs=+-|
  Sum1 : Sum  Inputs=+|+
  Sum2 : Sum  Inputs=+-|
  Sum3 : Sum  Inputs=|++
  Sum4 : Sum  Inputs=|++
  Switch : Switch  Criteria=u2 ~= 0  SaturateOnIntegerOverflow=off  InputSameDT=off
  Fhw : Outport
  wires:
  l/1 -> Sum/1, Relational Operator/1
  Constant4/1 -> Switch/1
  dlh/dt/1 -> Sum2/2
  Sum/1 -> Gain/1
  Product2/1 -> Sum1/2
  Sum1/1 -> Product4/2
  Gain/1 -> Product1/2
  Product3/1 -> Product2/1
  Sum4/1 -> Divide/2
  Sum2/1 -> Gain1/1
  Divide/1 -> Product1/1
  Product1/1 -> Sum1/1
  dl/dt/1 -> Sum2/1
  Constant/1 -> Product3/2
  Sum3/1 -> Product3/1
  Gain3/1 -> Sum4/1
  Ih/1 -> Gain2/1, Sum/2, Relational Operator/2, Gain3/1
  Constant1/1 -> Sum3/2
  Constant3/1 -> Sum4/2
  Relational Operator/1 -> Switch/2
  Switch/1 -> Product4/1
  Constant2/1 -> Divide/1
  Gain1/1 -> Product2/2
  Gain2/1 -> Sum3/1
  Constant5/1 -> Switch/3
  Product4/1 -> Fhw/1

== system PLANTA_CONTROL_OBS/PLANTA/Traslacion del carro ==
  F_tw : Inport
  F_hw : Inport  Port=2
  theta_l : Inport  Port=3
  Gain : Gain  Gain=2
  Gain1 : Gain  Gain=bt
  Gain2 : Gain  Gain=1/Mt
  Integrator : Integrator  InitialCondition=dx_t_ini
  Integrator1 : Integrator  InitialCondition=x_t_ini
  Product : Product
  Sin : Trigonometry
  Sum : Sum  Inputs=++-
  x_t : Outport
  dx_t : Outport  Port=2
  wires:
  Gain1/1 -> Sum/3
  Integrator1/1 -> x_t/1
  theta_l/1 -> Sin/1
  Sin/1 -> Product/2
  Sum/1 -> Gain2/1
  F_tw/1 -> Sum/1
  F_hw/1 -> Product/1
  Gain/1 -> Sum/2
  Integrator/1 -> dx_t/1, Gain1/1, Integrator1/1
  Product/1 -> Gain/1
  Gain2/1 -> Integrator/1  "ddx_t"

== system PLANTA_CONTROL_OBS/Nivel 2 - Control Regulatorio + Obs/Observador_Control_Posicion/Fuerzas de tension de cable en Carro ==
  x_td : Inport
  dx_td : Inport  Port=2
  x_t : Inport  Port=3
  dx_t : Inport  Port=4
  Add : Sum  Inputs=+-
  Add1 : Sum  Inputs=+-
  Add2 : Sum
  Gain : Gain  Gain=Ktw
  Gain1 : Gain  Gain=btw
  F_tw : Outport
  wires:
  Add1/1 -> Gain1/1
  Add/1 -> Gain/1
  Gain1/1 -> Add2/2
  x_td/1 -> Add/1
  dx_t/1 -> Add1/2
  dx_td/1 -> Add1/1
  Gain/1 -> Add2/1
  Add2/1 -> F_tw/1
  x_t/1 -> Add/2

== system PLANTA_CONTROL_OBS/Nivel 2 - Control Regulatorio + Obs/Observador_Control_Posicion/Observador ==
  x_td : Inport
  T_tm* : Inport  Port=2
  Discrete-Time Integrator : DiscreteIntegrator  InitialCondition=x_td_ini  SampleTime=T_s2  ICPrevOutput=DiscIntNeverNeededParam  ICPrevScaledInput=DiscIntNeverNeededParam
  Discrete-Time Integrator1 : DiscreteIntegrator  InitialCondition=dx_td_ini  SampleTime=T_s2  ICPrevOutput=DiscIntNeverNeededParam  ICPrevScaledInput=DiscIntNeverNeededParam
  Gain : Gain  Gain=rtd/(Jtd+Jtm_tb*(it)^2)
  Gain1 : Gain  Gain=Ke_tita
  Gain2 : Gain  Gain=Ke_w
  Gain3 : Gain  Gain=it
  Scope : Scope  NumInputPorts=3
  Sum1 : Sum  Inputs=|++
  Sum2 : Sum  Inputs=|++
  Sum3 : Sum  Inputs=+-|
  dx_td_obs : Outport
  wires:
  T_tm*/1 -> Gain3/1
  Gain/1 -> Sum1/1
  Sum1/1 -> Discrete-Time Integrator1/1  "ddx_td_obs"
  x_td/1 -> Scope/1, Sum3/1
  Sum3/1 -> Gain2/1, Gain1/1
  Gain1/1 -> Sum2/2
  Gain2/1 -> Sum1/2
  Sum2/1 -> Scope/3, Discrete-Time Integrator/1, dx_td_obs/1
  Gain3/1 -> Gain/1
  Discrete-Time Integrator/1 -> Scope/2, Sum3/2
  Discrete-Time Integrator1/1 -> Sum2/1

== system PLANTA_CONTROL_OBS/Nivel 2 - Control Regulatorio + Obs/Observador_Control_Posicion/Subsystem ==
  xt_obs : Inport
  xt_ref : Inport  Port=2
  Discrete Derivative : simulink/Discrete/Discrete Derivative  gainval=1.0  ICPrevScaledInput=0.0  OutMin=[]  OutMax=[]  OutDataType=fixdt(1, 16)  OutScaling=2^-10  DoSatur=off
  Gain : Gain  Gain=kp_pos
  Gain1 : Gain  Gain=kp_w
  Sum : Sum  Inputs=|++
  Sum1 : Sum  Inputs=|-+
  dxt_pos : Outport
  wires:
  xt_ref/1 -> Sum1/2
  Sum1/1 -> Discrete Derivative/1, Gain/1
  Gain/1 -> Sum/1  "dxt_pos"
  Gain1/1 -> Sum/2  "dxt_pos"
  Sum/1 -> dxt_pos/1
  xt_obs/1 -> Sum1/1
  Discrete Derivative/1 -> Gain1/1

== system PLANTA_CONTROL_OBS/Nivel 2 - Control Regulatorio + Obs/Observador_Control_Posicion/Traslacion del carro ==
  F_tw : Inport
  F_hw : Inport  Port=2
  theta_l : Inport  Port=3
  Discrete-Time Integrator : DiscreteIntegrator  InitialCondition=dx_t_ini  SampleTime=T_s2  ICPrevOutput=DiscIntNeverNeededParam  ICPrevScaledInput=DiscIntNeverNeededParam
  Discrete-Time Integrator1 : DiscreteIntegrator  InitialCondition=x_t_ini  SampleTime=T_s2  ICPrevOutput=DiscIntNeverNeededParam  ICPrevScaledInput=DiscIntNeverNeededParam
  Gain : Gain  Gain=2
  Gain1 : Gain  Gain=bt
  Gain2 : Gain  Gain=1/Mt
  Product : Product
  Sin : Trigonometry
  Sum : Sum  Inputs=++-
  x_t : Outport
  dx_t : Outport  Port=2
  wires:
  Gain1/1 -> Sum/3
  theta_l/1 -> Sin/1
  Sin/1 -> Product/2
  Sum/1 -> Gain2/1
  F_tw/1 -> Sum/1
  F_hw/1 -> Product/1
  Gain/1 -> Sum/2
  Product/1 -> Gain/1
  Gain2/1 -> Discrete-Time Integrator/1  "ddx_t"
  Discrete-Time Integrator/1 -> Discrete-Time Integrator1/1, Gain1/1, dx_t/1
  Discrete-Time Integrator1/1 -> x_t/1

== system PLANTA_CONTROL_OBS/PLANTA/Accionamiento de Izaje/Freno ==
  w_hm : Inport
  BRK_h : Inport  Port=2
  Constant : Constant  Value=0
  Gain5 : Gain  Gain=-bhd
  Saturation : Saturate  UpperLimit=Thb_Max  LowerLimit=-Thb_Max
  Scope : Scope
  Switch : Switch  Criteria=u2 > Threshold  SaturateOnIntegerOverflow=off  InputSameDT=off
  T_hb : Outport
  wires:
  Gain5/1 -> Saturation/1
  BRK_h/1 -> Switch/2
  Saturation/1 -> Switch/3
  Constant/1 -> Switch/1
  w_hm/1 -> Gain5/1
  Switch/1 -> Scope/1, T_hb/1

== system PLANTA_CONTROL_OBS/PLANTA/Accionamiento de Izaje/Freno Emergencia ==
  w_hd : Inport
  BRK_hE : Inport  Port=2
  Constant : Constant  Value=0
  Gain5 : Gain  Gain=-bhEb
  Saturation : Saturate  UpperLimit=ThEb_Max  LowerLimit=-ThEb_Max
  Switch : Switch  Criteria=u2 > Threshold  SaturateOnIntegerOverflow=off  InputSameDT=off
  T_hEB : Outport
  wires:
  Gain5/1 -> Saturation/1
  BRK_hE/1 -> Switch/2
  Saturation/1 -> Switch/3
  Constant/1 -> Switch/1
  w_hd/1 -> Gain5/1
  Switch/1 -> T_hEB/1

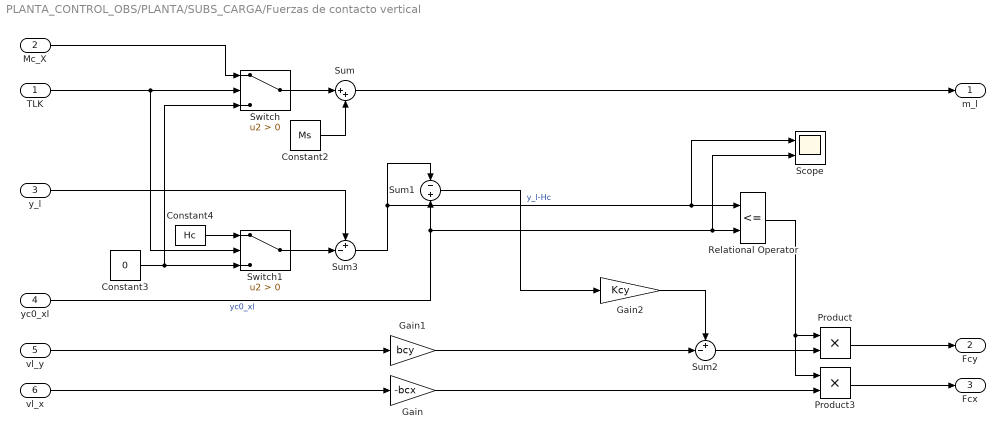
== system PLANTA_CONTROL_OBS/PLANTA/SUBS_CARGA/Fuerzas de contacto vertical ==
  TLK : Inport
  Mc_X : Inport  Port=2
  y_l : Inport  Port=3
  yc0_xl : Inport  Port=4
  vl_y : Inport  Port=5
  vl_x : Inport  Port=6
  Constant2 : Constant  Value=Ms
  Constant3 : Constant  Value=0
  Constant4 : Constant  Value=Hc
  Gain : Gain  Gain=-bcx
  Gain1 : Gain  Gain=bcy
  Gain2 : Gain  Gain=Kcy
  Product : Product
  Product3 : Product
  Relational Operator : RelationalOperator  Operator=<=  OutDataTypeStr=boolean  RndMeth=Simplest  InputSameDT=off
  Scope : Scope  NumInputPorts=2
  Sum : Sum  Inputs=|++
  Sum1 : Sum  Inputs=-|+
  Sum2 : Sum  Inputs=+-|
  Sum3 : Sum  Inputs=+-|
  Switch : Switch  Criteria=u2 > Threshold  SaturateOnIntegerOverflow=off  InputSameDT=off
  Switch1 : Switch  Criteria=u2 > Threshold  SaturateOnIntegerOverflow=off  InputSameDT=off
  m_l : Outport
  Fcy : Outport  Port=2
  Fcx : Outport  Port=3
  wires:
  TLK/1 -> Switch/2, Switch1/2
  Gain1/1 -> Sum2/2
  Switch/1 -> Sum/1
  Constant3/1 -> Switch1/3, Switch/3
  yc0_xl/1 -> Scope/2, Relational Operator/2, Sum1/2  "yc0_xl"
  Constant2/1 -> Sum/2
  Sum3/1 -> Scope/1, Relational Operator/1, Sum1/1  "y_l-Hc"
  Sum2/1 -> Product/2
  vl_y/1 -> Gain1/1
  Gain/1 -> Product3/2
  Switch1/1 -> Sum3/2
  Constant4/1 -> Switch1/1
  vl_x/1 -> Gain/1
  Gain2/1 -> Sum2/1
  Sum1/1 -> Gain2/1
  Sum/1 -> m_l/1
  y_l/1 -> Sum3/1
  Mc_X/1 -> Switch/1
  Product/1 -> Fcy/1
  Product3/1 -> Fcx/1
  Relational Operator/1 -> Product3/1, Product/1

== matlab function PLANTA_CONTROL_OBS/PLANTA/PERFIL_OBSTACULOS/sensor ==
  data: y0_array input; distancia output; index input; Yt0 parameter
function distancia= mideDistancia(y0_array,index, Yt0)
distancia = Yt0-y0_array(index);

== matlab function PLANTA_CONTROL_OBS/PLANTA/Altura perfil obstaculos (A partir de posicion x_l)/Calculo ==
  data: y0_array input; yc0_xt output; index input
function yc0_xt= calcula_y0(y0_array,index)

if (index>0 && index<=32)
    yc0_xt =y0_array(index);
else
    yc0_xt=0;    
end
